simulink subsystem "Tracker"  (R2024a)
settings: Solver=VariableStepAuto  StartTime=0.0  StopTime=10.0  RelTol=1e-3
undefined symbols (not defined in the file): M, N, sceneOrigin, Ts
libraries: drivinglib x1
settings Model: Creator=L03509110  LastModifiedBy=L03509110

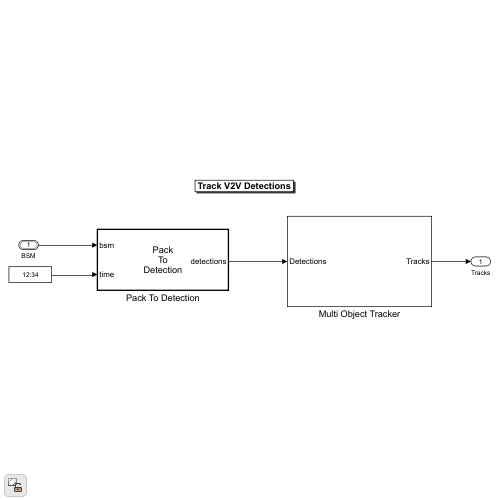
[thumbnail: Simulink's stored preview of the top-level diagram]
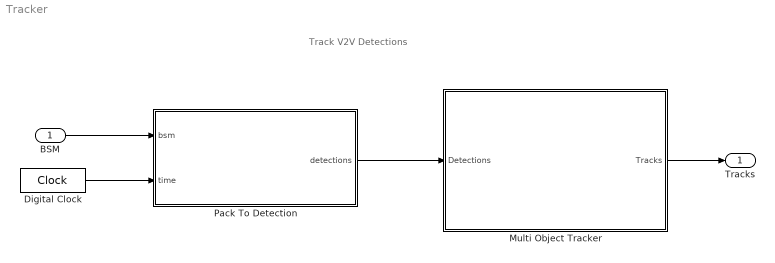
== system Tracker ==
  note: Track V2V Detections
  BSM : Inport  OutDataTypeStr=Bus: BusBSM  SampleTime=Ts
  Digital Clock : DigitalClock  SampleTime=Ts
  Multi Object Tracker : Subsystem
  Pack To Detection : MATLAB Function  TreatAsAtomicUnit=on  mask{origin=sceneOrigin, outputStruct=Simulink.Bus.createMATLABStruct('BusTargetDetections')}
      mask prompts: origin "Scene Origin"; outputStruct "Output Struct"
  Tracks : Outport
  wires:
  BSM/1 -> Pack To Detection/1(bsm)
  Pack To Detection/1(detections) -> Multi Object Tracker/1(Detections)
  Multi Object Tracker/1(Tracks) -> Tracks/1
  Digital Clock/1 -> Pack To Detection/2(time)

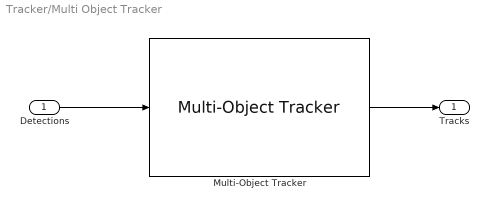
== system Tracker/Multi Object Tracker ==
  Detections : Inport  OutDataTypeStr=Bus: BusTargetDetections
  Multi-Object Tracker : drivinglib/Multi-Object Tracker  TrackerIndex=uint32( 0 )  FilterInitializationFcn=initcaekf  AssignmentThreshold=assignThresh  ConfirmationThreshold=[M N]  DeletionThreshold=[ 5, 5 ]  MaxNumTracks=numTracks  MaxNumSensors=numSensors  OOSMHandling=Terminate  StateParametersSimulink=struct  HasStateParametersInput=off  TimeInputSource=Auto  HasCostMatrixInput=off  HasDetectableTrackIDsInput=off  BusNameSource=Property  BusName=BusMultiObjectTracker  TentativeTracksOutputPort=off  AllTracksOutputPort=off  SimulateUsing=Interpreted execution
  Tracks : Outport
  wires:
  Detections/1 -> Multi-Object Tracker/1
  Multi-Object Tracker/1 -> Tracks/1

== matlab function Tracker/Pack To Detection ==
  data: bsm input Bus: BusBSM; detections output Bus: BusTargetDetections; origin parameter; outputStruct parameter; time input
function detections = packToDetection(bsm,origin, outputStruct, time)

detections = outputStruct; 
if bsm.NumOfBSM>0
    detections.NumDetections = bsm.NumOfBSM;
    measCov = cast(diag([1,1,1,1,1,1]),'double');
    measparms = struct('Frame',drivingCoordinateFrameType(1),...
        'OriginPosition',zeros(3,1,'double'),...
        'Orientation',eye(3,'double'),...
        'HasVelocity',true, ...
        'HasElevation',false);

    for idx = 1:bsm.NumOfBSM        
        BSMCoreData = bsm.BSMCoreData(idx);
        
        lla = [double(BSMCoreData.Lattitude)*10^-7,...
            double(BSMCoreData.Longitude)*10^-7,...
            double(BSMCoreData.Elevation)*0.1];
        
        % Transform geodetic coordinates to local east-north-up coordinates

        pos = [0 0 0];
        [pos(1),pos(2),pos(3)] = latlon2local(lla(1),lla(2),lla(3),origin);
        speed = double(BSMCoreData.Speed)*0.02;
        heading = double(BSMCoreData.Heading)*0.0125;
        vy = speed*cosd(heading);
        vx = speed*sind(heading);
        
        detections.Detections(idx).Time = time;double(BSMCoreData.SecMark)*1e-3;
        detections.Detections(idx).Measurement = [pos(1); pos(2); 0; vx; vy; 0]; % [x;y;z;vx;vy;vz]
        detections.Detections(idx).MeasurementNoise = measCov;
        detections.Detections(idx).SensorIndex = 1;
        detections.Detections(idx).ObjectClassID = 1;
        detections.Detections(idx).MeasurementParameters = measparms;
    end
end

end
